simulink model "BuckyWagon_01"  (Simulink 7.5)
settings: Solver=FixedStepDiscrete  StartTime=0.0  StopTime=10.0  RelTol=1e-3
PreLoadFcn:
  | try, eval([bdroot '_setup']); catch, eval('model_setup', ''); end
InitFcn:
  | try, eval([bdroot '_setup']); catch, eval('model_setup', ''); end
undefined symbols (not defined in the file): ECU565, High, Low, miniviewSetup, motohawk_build_version, motohawk_get_faults, motohawk_setup_toolchains, motohawk_trunc_name, motohawk_vardec_config_group, motohawk_vardec_path, tc, True
libraries: MotoHawk_lib x381, simulink x26, miniview_lib x10, motohawk_control_primitives_lib x8, motohawk_engine_lib x6, motohawk_annotations_lib x2
(part 6 of 6)

== system BuckyWagon_01/Strategy/MiniViewDisplay/Send String_efficient/Subsystem ==
  string # : Inport  OutDataType=sfix(16)  OutScaling=2^0
  string : Inport  Port=2  OutDataType=sfix(16)  OutScaling=2^0
  Trigger : TriggerPort  TriggerType=function-call
  Demux3 : Demux  Outputs=[7 7 3 1]
  Function-Call Generator : simulink/Ports & Subsystems/Function-Call Generator  sample_time=-1  numberOfIterations=1
  Function-Call Subsystem : Subsystem  TreatAsAtomicUnit=on
  Function-Call Subsystem1 : Subsystem  TreatAsAtomicUnit=on
  Send Substring (page 0) : miniview_lib/Send Substring (page 0)  SystemSampleTime=-1  miniview_CAN_channel=miniview_CAN_channel
  Send Substring (page 1) : miniview_lib/Send Substring (page 1)  SystemSampleTime=-1  miniview_CAN_channel=miniview_CAN_channel
  Send Substring (page 2) : miniview_lib/Send Substring (page 2)  SystemSampleTime=-1  miniview_CAN_channel=miniview_CAN_channel
  Terminator : Terminator
  Terminator1 : Terminator
  wires:
  Demux3/3 -> Send Substring (page 2)/2
  Demux3/2 -> Send Substring (page 1)/2, Function-Call Subsystem1/1(In1)
  Demux3/1 -> Send Substring (page 0)/2, Function-Call Subsystem/1(In1)
  string/1 -> Demux3/1  "string"
  string #/1 -> Send Substring (page 1)/1, Send Substring (page 2)/1, Send Substring (page 0)/1  "string #"
  Function-Call Generator/1 -> Send Substring (page 0)/Trigger
  Send Substring (page 0)/1 -> Function-Call Subsystem/Trigger
  Function-Call Subsystem/1(Out) -> Send Substring (page 1)/Trigger
  Send Substring (page 1)/1 -> Function-Call Subsystem1/Trigger
  Function-Call Subsystem1/1(Out) -> Send Substring (page 2)/Trigger
  Demux3/4 -> Terminator/1
  Send Substring (page 2)/1 -> Terminator1/1

== system BuckyWagon_01/Strategy/MiniViewDisplay/Up Button/Subsystem ==
  Trigger : TriggerPort  TriggerType=function-call
  Read CAN Message : MotoHawk_lib/CAN Blocks/Read CAN Message  nam=['CAN_' num2str(miniview_CAN_channel)]  bus=-2  msg=miniview_button_up  queue=1  slot='miniview_button_up'  valid=off  stale=off  labelwires=on
  Signal Specification : SignalSpecification  DataType=boolean  OutDataType=sfix(16)  OutScaling=2^0  OutDataTypeStr=boolean
  Signal Specification1 : SignalSpecification  DataType=uint8  OutDataType=sfix(16)  OutScaling=2^0  OutDataTypeStr=uint8
  Up Asserted : Outport  OutDataType=sfix(16)  OutScaling=2^0
  Up Count : Outport  Port=2  OutDataType=sfix(16)  OutScaling=2^0
  wires:
  Signal Specification1/1 -> Up Count/1  "up count"
  Signal Specification/1 -> Up Asserted/1  "up asserted"
  Read CAN Message/2 -> Signal Specification1/1  "up count"
  Read CAN Message/1 -> Signal Specification/1  "up asserted"

== system BuckyWagon_01/Strategy/Sensors/Brusa Charger/PluggedInDetect ==
  MainsVolt : Inport  OutDataType=sfix(16)  OutScaling=2^0
  Thres : Inport  Port=2  OutDataType=sfix(16)  OutScaling=2^0
  Time : Inport  Port=3  OutDataType=sfix(16)  OutScaling=2^0
  Chart : Stateflow chart  TreatAsAtomicUnit=on
  Relational Operator : RelationalOperator  Operator=>  LogicOutDataTypeMode=boolean  OutDataTypeStr=boolean
  pluggedIn : Outport  OutDataType=sfix(16)  OutScaling=2^0
  wires:
  MainsVolt/1 -> Relational Operator/1
  Thres/1 -> Relational Operator/2
  Chart/1(pluggedIn) -> pluggedIn/1
  Relational Operator/1 -> Chart/2(mainsOn)
  Time/1 -> Chart/1(histTime)

== system BuckyWagon_01/Strategy/Sensors/Linear Sensor Characterization/If Action Subsystem ==
  In : Inport  OutDataType=sfix(16)  OutScaling=2^0
  Action Port : ActionPort  ActionType=then
  Out : Outport  OutDataType=sfix(16)  OutScaling=2^0
  wires:
  In/1 -> Out/1

== system BuckyWagon_01/Strategy/Sensors/Linear Sensor Characterization/If Action Subsystem1 ==
  In : Inport  OutDataType=sfix(16)  OutScaling=2^0
  Action Port : ActionPort  ActionType=elseif
  Out : Outport  OutDataType=sfix(16)  OutScaling=2^0
  wires:
  In/1 -> Out/1

== system BuckyWagon_01/Strategy/Sensors/Linear Sensor Characterization/If Action Subsystem2 ==
  In : Inport  OutDataType=sfix(16)  OutScaling=2^0
  Action Port : ActionPort  ActionType=else
  Out : Outport  OutDataType=sfix(16)  OutScaling=2^0
  wires:
  In/1 -> Out/1

== system BuckyWagon_01/Strategy/Control Strategy/Assist/StallTorqueFault/Hysterisis ==
  HiThresh : Inport  OutDataType=sfix(16)  OutScaling=2^0
  LowThresh : Inport  Port=2  OutDataType=sfix(16)  OutScaling=2^0
  Signal : Inport  Port=3  OutDataType=sfix(16)  OutScaling=2^0
  Hysteresis : Subsystem
  LT : RelationalOperator  ZeroCross=off  InputSameDT=on
  LT1 : RelationalOperator  Operator=<=  ZeroCross=off  InputSameDT=on
  Threshold : Outport  OutDataType=sfix(16)  OutScaling=2^0
  wires:
  LT/1 -> Hysteresis/1(Hi)  "AboveHiTarget"
  LT1/1 -> Hysteresis/2(Lo)  "BelowLoTarget"
  Hysteresis/1("Out (Lo=0, Hi=1)") -> Threshold/1
  HiThresh/1 -> LT/2
  LowThresh/1 -> LT1/2
  Signal/1 -> LT/1, LT1/1

== system BuckyWagon_01/Strategy/Control Strategy/HV Controller/Contacter Controller/Delay ==
  note: Delay the rising and falling of a boolean signal
  In : Inport  OutDataType=sfix(16)  OutScaling=2^0
  Constant1 : Constant  Value=0  OutDataType=sfix(16)  OutScaling=2^0  OutDataTypeStr=Inherit: Inherit via back propagation
  Constant3 : Constant  Value=0  OutDataType=sfix(16)  OutScaling=2^0  OutDataTypeStr=Inherit: Inherit via back propagation
  Data Type Conversion : DataTypeConversion  OutDataType=sfix(16)  OutScaling=2^0  RndMeth=Zero
  Data Type Conversion1 : DataTypeConversion  OutDataType=sfix(16)  OutScaling=2^0  RndMeth=Zero
  Logical Operator : Logic  Operator=NOT  OutDataTypeMode=boolean  OutDataTypeStr=boolean
  Logical Operator1 : Logic  OutDataTypeMode=boolean  OutDataTypeStr=boolean
  Logical Operator2 : Logic  OutDataTypeMode=boolean  OutDataTypeStr=boolean
  MotoHawk S-R Flip-Flop : Subsystem  mask(MotoHawk S-R Flip-Flop){ic_bool=false}
      mask prompts: ic_bool "Initial condition Q (boolean)"
      mask help:
      | When input S (set) is TRUE, output Q is TRUE (and latched until reset).
      | When input R (reset) is TRUE, output Q is FALSE (and latched until set).
      | If both inputs S and R are TRUE, output Q is FALSE (reset wins).
      mask Display:
      | patch([0 0 1 1], [0 0.075 0.075 0], [230/255 0/255 0/255])
      | patch([0 0 1 1], [0.025 0.05 0.05 0.025], [150/255 0/255 0/255])
      | patch([0 0 1 1], [0 0.025 0.025 0], [0/255 0/255 0/255])
  Relational Operator1 : RelationalOperator  LogicOutDataTypeMode=boolean  OutDataTypeStr=boolean  ZeroCross=off  InputSameDT=on
  Relational Operator2 : RelationalOperator  LogicOutDataTypeMode=boolean  OutDataTypeStr=boolean  ZeroCross=off  InputSameDT=on
  Sum : Sum  Inputs=++|  OutDataType=sfix(16)  OutScaling=2^0  RndMeth=Zero  SaturateOnIntegerOverflow=on  InputSameDT=on
  Sum1 : Sum  Inputs=++|  OutDataType=sfix(16)  OutScaling=2^0  RndMeth=Zero  SaturateOnIntegerOverflow=on  InputSameDT=on
  Switch : Switch  Criteria=u2 ~= 0  Threshold=1  RndMeth=Zero  ZeroCross=off  InputSameDT=on
  Switch1 : Switch  Criteria=u2 ~= 0  Threshold=1  RndMeth=Zero  ZeroCross=off  InputSameDT=on
  Terminator : Terminator
  Unit Delay : UnitDelay  SampleTime=-1
  Unit Delay1 : UnitDelay  SampleTime=-1
  off delay : Constant  Value=10  OutDataType=sfix(16)  OutScaling=2^0
  on delay : Constant  Value=0  OutDataType=sfix(16)  OutScaling=2^0
  Out : Outport  OutDataType=sfix(16)  OutScaling=2^0
  wires:
  Logical Operator1/1 -> MotoHawk S-R Flip-Flop/2(R)
  Logical Operator2/1 -> MotoHawk S-R Flip-Flop/1(S)
  Relational Operator1/1 -> Logical Operator2/2
  Relational Operator2/1 -> Logical Operator1/2
  MotoHawk S-R Flip-Flop/2(!Q) -> Terminator/1
  MotoHawk S-R Flip-Flop/1(Q) -> Out/1
  off delay/1 -> Relational Operator2/2
  Logical Operator/1 -> Logical Operator1/1, Switch1/2, Data Type Conversion1/1
  Data Type Conversion1/1 -> Sum1/2  "0 to 1"
  Sum1/1 -> Switch1/1  "0 to 65535 (saturate hi)"
  Constant3/1 -> Switch1/3
  Switch1/1 -> Relational Operator2/1, Unit Delay1/1  "0 to 65535"
  In/1 -> Logical Operator/1, Logical Operator2/1, Switch/2, Data Type Conversion/1
  Data Type Conversion/1 -> Sum/2  "0 to 1"
  Sum/1 -> Switch/1  "0 to 65535 (saturate hi)"
  Constant1/1 -> Switch/3
  Switch/1 -> Unit Delay/1, Relational Operator1/1  "0 to 65535"
  on delay/1 -> Relational Operator1/2
  Unit Delay1/1 -> Sum1/1  "0 to 65535"
  Unit Delay/1 -> Sum/1  "0 to 65535"

== system BuckyWagon_01/Strategy/MiniViewDisplay/Send String_efficient/Subsystem/Function-Call Subsystem ==
  In1 : Inport  OutDataType=sfix(16)  OutScaling=2^0
  function : TriggerPort  TriggerType=function-call
  Compare To Zero : simulink/Logic and Bit Operations/Compare To Zero  SystemSampleTime=-1  relop=~=  LogicOutDataTypeMode=uint8  ZeroCross=off
  Enabled Subsystem : Subsystem  TreatAsAtomicUnit=on
  Logical Operator : Logic  Inputs=1  AllPortsSameDT=off  OutDataTypeMode=boolean  OutDataTypeStr=boolean
  Out : Outport  OutDataType=sfix(16)  OutScaling=2^0
  wires:
  Compare To Zero/1 -> Logical Operator/1
  In1/1 -> Compare To Zero/1
  Logical Operator/1 -> Enabled Subsystem/Enable
  Enabled Subsystem/1(Out1) -> Out/1

== system BuckyWagon_01/Strategy/MiniViewDisplay/Send String_efficient/Subsystem/Function-Call Subsystem1 ==
  In1 : Inport  OutDataType=sfix(16)  OutScaling=2^0
  function : TriggerPort  TriggerType=function-call
  Compare To Zero : simulink/Logic and Bit Operations/Compare To Zero  SystemSampleTime=-1  relop=~=  LogicOutDataTypeMode=uint8  ZeroCross=off
  Enabled Subsystem : Subsystem  TreatAsAtomicUnit=on
  Logical Operator : Logic  Inputs=1  AllPortsSameDT=off  OutDataTypeMode=boolean  OutDataTypeStr=boolean
  Out : Outport  OutDataType=sfix(16)  OutScaling=2^0
  wires:
  Enabled Subsystem/1(Out1) -> Out/1
  Logical Operator/1 -> Enabled Subsystem/Enable
  In1/1 -> Compare To Zero/1
  Compare To Zero/1 -> Logical Operator/1

== system BuckyWagon_01/Strategy/Control Strategy/Assist/StallTorqueFault/Hysterisis/Hysteresis ==
  note: Hi & !Lo => Hi
      | Lo & !Hi => Lo
      | Otherwise, Hold
  Hi : Inport  OutDataType=sfix(16)  OutScaling=2^0
  Lo : Inport  Port=2  OutDataType=sfix(16)  OutScaling=2^0
  Combinatorial  Logic : CombinatorialLogic  TruthTable=[0 0;0 1;1 1;0 0]
  Demux : Demux  Outputs=2
  Mux : Mux  Inputs=2
  Switch1 : Switch  Threshold=0.5  SaturateOnIntegerOverflow=on  InputSameDT=on
  Unit Delay : UnitDelay  SampleTime=-1
  "Out (Lo=0, Hi=1)" : Outport  OutDataType=sfix(16)  OutScaling=2^0
  wires:
  Mux/1 -> Combinatorial  Logic/1
  Combinatorial  Logic/1 -> Demux/1
  Demux/1 -> Switch1/1
  Demux/2 -> Switch1/2
  Unit Delay/1 -> Switch1/3
  Switch1/1 -> Unit Delay/1, "Out (Lo=0, Hi=1)"/1
  Hi/1 -> Mux/1
  Lo/1 -> Mux/2

== system BuckyWagon_01/Strategy/Control Strategy/HV Controller/Contacter Controller/Delay/MotoHawk S-R Flip-Flop ==
  note: MotoHawk S-R Flip-Flop
  S : Inport  OutDataType=sfix(16)  OutScaling=2^0
  R : Inport  Port=2  OutDataType=sfix(16)  OutScaling=2^0
  Logical Operator : Logic  Operator=OR  OutDataTypeMode=boolean  OutDataTypeStr=boolean
  Logical Operator1 : Logic  Operator=NOT  OutDataTypeMode=boolean  OutDataTypeStr=boolean
  Logical Operator2 : Logic  OutDataTypeMode=boolean  OutDataTypeStr=boolean
  Logical Operator3 : Logic  Operator=NOT  OutDataTypeMode=boolean  OutDataTypeStr=boolean
  Signal Specification : SignalSpecification  DataType=boolean  OutDataType=sfix(16)  OutScaling=2^0  OutDataTypeStr=boolean
  Signal Specification1 : SignalSpecification  DataType=boolean  OutDataType=sfix(16)  OutScaling=2^0  OutDataTypeStr=boolean
  Unit Delay : UnitDelay  X0=ic_bool  SampleTime=-1
  Q : Outport  OutDataType=sfix(16)  OutScaling=2^0
  !Q : Outport  Port=2  OutDataType=sfix(16)  OutScaling=2^0
  wires:
  Logical Operator3/1 -> !Q/1
  R/1 -> Signal Specification/1
  S/1 -> Signal Specification1/1
  Signal Specification1/1 -> Logical Operator/2
  Signal Specification/1 -> Logical Operator1/1
  Logical Operator2/1 -> Q/1, Unit Delay/1, Logical Operator3/1
  Unit Delay/1 -> Logical Operator/1
  Logical Operator/1 -> Logical Operator2/1
  Logical Operator1/1 -> Logical Operator2/2

== system BuckyWagon_01/Strategy/MiniViewDisplay/Send String_efficient/Subsystem/Function-Call Subsystem/Enabled Subsystem ==
  Enable : EnablePort
  Function-Call Generator : simulink/Ports & Subsystems/Function-Call Generator  sample_time=-1  numberOfIterations=1
  Out1 : Outport  OutDataType=sfix(16)  OutScaling=2^0
  wires:
  Function-Call Generator/1 -> Out1/1

== system BuckyWagon_01/Strategy/MiniViewDisplay/Send String_efficient/Subsystem/Function-Call Subsystem1/Enabled Subsystem ==
  Enable : EnablePort
  Function-Call Generator : simulink/Ports & Subsystems/Function-Call Generator  sample_time=-1  numberOfIterations=1
  Out1 : Outport  OutDataType=sfix(16)  OutScaling=2^0
  wires:
  Function-Call Generator/1 -> Out1/1

== stateflow chart Strategy/Control Strategy/Reverse/Chart ==
  state Main
    state ButtonDebounce [parallel]
      settings: executionOrder=1
      state waitRelease
        entry:buttonPress;
      state TransistionOn
        during:timer++;
      state TransistionOff
        during:timer++;
      TransistionOff -> TransistionOff [order 2] : [revButton]
          | {timer = 0;}
      TransistionOff -> TransistionOn [order 1] : [timer >= offTime]
      TransistionOn -> waitRelease [order 2] : [timer >= onTime]
      waitRelease -> TransistionOff : [~revButton]
      TransistionOn -> TransistionOn [order 1] : [~revButton]
          | {timer = 0;}
      (default) -> TransistionOn
    state ReverseLogic [parallel]
      settings: executionOrder=2
      state Forward
        entry:inReverse = 0;
      state Reverse
        entry:inReverse = 1;
      Reverse -> Forward : buttonPress...
          | [(speed < fwdSpdThres)&&...
          | (accel < fwdAccThres)]
      Forward -> Reverse : buttonPress...
          | [(speed < revSpdThres)&&...
          | (accel < revAccThres)]
      (default) -> Forward
  data: accel input double; speed input double; revButton input double; fwdAccThres input double; fwdSpdThres input double; inReverse output double; offTime input double; revAccThres input double; revSpdThres input double; timer local double; onTime input double
  events: buttonPress local EITHER_EDGE_EVENT

== stateflow chart Strategy/MiniViewDisplay/Chart ==
  state List
    state List_Wait
    state List_Wait2
    state List_Idle
      entry:
      stringNum = 0;
    state List_Init
      entry:
      clearScreen;
      //draw lines and name
      stringNum = 15;
      sprintf(charPtr(&string[0]), "UWMAD");
      string[5] = 0;
      sendString;
      y0 = 8;
      x0 = 0;
      x1 = 63;
      lineColor = BLACK;
      fillColor = WHITE;
      drawHLine;
      y0 = 54;
      drawHLine;
      hCenter = 1;
      vCenter = 0;
      font = FONT4x6;
      x0 = 32;
      y0 = 2;
      drawString;
      listIndexO = listIndex;
    (junction 83) -> (junction 93) [order 1] : [statusTxtMode == 1]...
        | {fillColor = BLACK; lineColor = BLACK;...
        | drawRect; lineColor = WHITE;}
    (junction 90) -> (junction 83) [order 2] : {y0 = 55; y1 = 63; x0 = 0; x1 = 63;...
        | memcpy(&string[0], &statusTxt[0], 9);...
        | string[9] = 0; sendString;}
    (junction 83) -> (junction 93) [order 2] : {lineColor = WHITE;...
        | drawRect;...
        | lineColor = BLACK;}
    List.List_Idle -> List.List_Idle [order 2] : tick /timer++;
    (junction 85) -> List.List_Idle : {timer = 0;}
    (junction 86) -> List.List_Idle [order 1] : [listIndex == 0]
    List.List_Idle -> (junction 86) [order 3] : upPressed
    (junction 86) -> (junction 87) [order 2] : {listIndexO = listIndex-1;...
        | writeListIndex;}
    List_Init -> (junction 87)
    List.List_Idle -> (junction 88) [order 4] : downPressed
    (junction 88) -> (junction 87) [order 2] : {listIndexO = listIndex+1;...
        | writeListIndex;;}
    (junction 88) -> List.List_Idle [order 1] : [listIndex == numFields-6]
    (junction 93) -> (junction 85) : {y0 = 56; font = FONT4x6; x0 = 17;...
        | drawString;}
    (junction 89) -> (junction 90) [order 2] : {sprintf(charPtr(&string[0]), "%-4d", data[stringNum+listIndex]);...
        | string[4] = 0; sendString;...
        | x0 = 42; x1 = 57; y0 = 12+stringNum*7; y1 = y0+6;...
        | lineColor = 0; drawRect; lineColor = 1
        | drawString;...
        |  oldData[stringNum] = data[stringNum+listIndex];...
        | stringNum++;}
    List.List_Idle -> (junction 90) [order 1] : tick [timer >= UPDATE_TIME]...
        | {stringNum = 0;...
        | fillColor = WHITE; hCenter = 0;}
    (junction 90) -> (junction 89) [order 1] : [stringNum < 6]
    (junction 87) -> (junction 91) : {stringNum = 0;}
    (junction 89) -> (junction 90) [order 1] : [oldData[stringNum] == data[stringNum+listIndex]]...
        | {stringNum++;}
    (junction 91) -> (junction 91) [order 1] : [stringNum < 6]...
        | {memcpy(&string[0], &names[10*(listIndexO+stringNum)], 10);...
        | sendString; stringNum++;}
    List_Wait2 -> (junction 90) : {stringNum = 0;}
    (junction 91) -> List_Wait [order 2]
    (junction 121) -> List_Init [order 2]
    (junction 92) -> List_Wait2 [order 2]
    List_Wait -> (junction 92) : {x0 = 9; y0 = 12; x1 = 41; y1 = 53;
        | lineColor = 0; fillColor = 0;
        | drawRect; lineColor = 1;
        | hCenter = 0; stringNum = 0;}
    (junction 121) -> (junction 121) [order 1] : [stringNum < 6]...
        | {oldData[stringNum] = ...
        | data[stringNum+listIndex]+1;...
        | stringNum++;}
    (junction 92) -> (junction 92) [order 1] : [stringNum < 6]...
        | {y0 = 12 + stringNum*7;...
        | drawString;stringNum++;}
    (default) -> (junction 121) : {stringNum = 0}
  state PowerupDelay
    entry:timer = 0;
    during:timer++;
  state Single
    state singleNames
      entry:
      hCenter = 1;
      font = FONT6x8;
      x0 = 30;
      stringNum = 0;
      memcpy(&string[0], &names[10*singleIndex], 10);
      sendString;
      y0 = 14;
      drawString;
    state Single_Init
      entry:
      clearScreen;
      //draw string
      stringNum = 15;
      sprintf(charPtr(&string[0]), "UWMAD");
      string[5] = 0;
      sendString;
      hCenter = 1;
      vCenter = 0;
      font = FONT4x6;
      x0 = 32; y0 = 2;
      lineColor = BLACK;
      fillColor = WHITE;
      drawString;
      //draw lines
      y0 = 8; x0 = 0; x1 = 64;
      drawHLine;
      y0 = 54;
      drawHLine;
      oldData[0] = data[singleIndex]+1
    state List_Idle
    (junction 76) -> (junction 74) : {y0 = 56; font = FONT4x6; x0 = 17;...
        | drawString;}
    (junction 117) -> (junction 118) [order 4] : [barGraphMode[singleIndex] == 3]...
        | {x0 = temp;...
        | drawVLine;}
    Single_Init -> singleNames
    (default) -> Single_Init
    (junction 75) -> (junction 76) [order 1] : [statusTxtMode == 1]...
        | {fillColor = BLACK; lineColor = BLACK;...
        | drawRect; lineColor = WHITE;}
    (junction 119) -> (junction 75) : {y0 = 55; y1 = 63; x0 = 0; x1 = 63;...
        | memcpy(&string[0], &statusTxt[0], 9);...
        | string[9] = 0; sendString;}
    (junction 120) -> (junction 119)
    (junction 74) -> Single.List_Idle : {timer = 0;}
    Single.List_Idle -> Single.List_Idle [order 2] : tick /timer++;
    (junction 115) -> (junction 119) [order 1] : [oldData[0] ==...
        |  data[singleIndex] ]
    (junction 118) -> (junction 120)
    (junction 117) -> (junction 118) [order 3] : [barGraphMode[singleIndex] == 1]...
        | {x0 = temp; fillColor = BLACK; drawRect;}
    (junction 116) -> (junction 117) [order 3] : {temp = (int32(data[singleIndex]) - barMin[singleIndex] )*52 /...
        |  (barMax[singleIndex]-barMin[singleIndex]) + 6;}
    (junction 117) -> (junction 118) [order 2] : [(barGraphMode[singleIndex] == 2) && (temp < 32)]...
        | {x0 = temp; x1 = 32; fillColor = BLACK; drawRect;}
    Single.List_Idle -> (junction 115) [order 1] : tick [timer >= UPDATE_TIME]...
        | {stringNum = 0;font = FONT8x15;...
        | fillColor = WHITE; hCenter = 0;}
    (junction 117) -> (junction 118) [order 5] : {x1 = temp; fillColor = BLACK; drawRect;}
    (junction 116) -> (junction 117) [order 2] : [data[singleIndex] <min(barMin[singleIndex], barMax[singleIndex])]...
        | {temp = ((min(barMin[singleIndex], barMax[singleIndex]) -...
        | barMin[singleIndex] )*52 / (barMax[singleIndex]-barMin[singleIndex])) + 6;}
    (junction 115) -> (junction 116) [order 2] : {sprintf(charPtr(&string[0]), "%4d", data[singleIndex]);...
        | sendString;...
        | x0 = 0; x1 = 64; y0 = 25; y1 = 39;fillColor = WHITE;...
        | lineColor = 0; drawRect; lineColor = BLACK; x0 = 15;...
        | drawString; oldData[0] = data[singleIndex];
        | x0 = 6; x1 = 58; y0 = 41; y1 = 48;
        | lineColor = BLACK; drawRect;}
    (junction 116) -> (junction 117) [order 1] : [data[singleIndex] > max(barMin[singleIndex], barMax[singleIndex])]...
        | {temp = ((max(barMin[singleIndex], barMax[singleIndex]) - ...
        | barMin[singleIndex] )*52 / (barMax[singleIndex]-barMin[singleIndex])) + 6;}
    (junction 117) -> (junction 118) [order 1] : [(barGraphMode[singleIndex] == 2) && (temp >= 32)]...
        | {x1 = temp; fillColor = BLACK; x0 = 32; drawRect;}
    singleNames -> Single.List_Idle : {timer = UPDATE_TIME;}
    (junction 75) -> (junction 76) [order 2] : {lineColor = WHITE;...
        | fillColor = WHITE;...
        | drawRect;...
        | lineColor = BLACK;}
  state Setup
    state wait
      entry:
      clearScreen;
      setupIndex = 0;
    state setup_Wait
    state setup_Idle
      entry:
      stringNum = 0;
    state Setup_Init
      entry:
      clearScreen;
      //draw lines and name
      stringNum = 15;
      sprintf(charPtr(&string[0]), "UWMAD");
      string[5] = 0;
      sendString;
      y0 = 8;
      x0 = 0;
      x1 = 63;
      lineColor = BLACK;
      fillColor = WHITE;
      drawHLine;
      y0 = 54;
      drawHLine;
      hCenter = 1;
      vCenter = 0;
      font = FONT4x6;
      x0 = 32;
      y0 = 2;
      drawString;
      setupVIndex = 0;
    state storeSelect [function]
      (junction 102) -> (junction 103) [order 1] : [setupIndex == 1]...
          | {singleIndexO = selectIndex; writeSingleIndex;}
      (default) -> (junction 102)
      (junction 102) -> (junction 103) [order 2] : [(setupIndex == 2) || (setupIndex == 3)]...
          | {dualIndexO = dualIndex;...
          | dualIndexO[setupIndex-2] = selectIndex;...
          | writeDualIndex;}
      (junction 102) -> (junction 103) [order 3] : [setupIndex >= 4]...
          | {quadIndexO = quadIndex;...
          | quadIndexO[setupIndex-4] = selectIndex;...
          |  writeQuadIndex;}
    state loadSelect [function]
      (junction 100) -> (junction 101) [order 1] : [setupIndex == 1]...
          | {selectIndex = singleIndex;}
      (default) -> (junction 100)
      (junction 100) -> (junction 101) [order 2] : [(setupIndex == 2) || (setupIndex == 3)]...
          | {selectIndex = dualIndex[setupIndex-2];}
      (junction 100) -> (junction 101) [order 3] : [setupIndex >= 4]...
          | {selectIndex = quadIndex[setupIndex-4];}
    state select_var
      state select_Wait
      state select_Idle
        entry:
      state Select_Init
        entry:
        clearScreen;
        //draw lines and name
        stringNum = 15;
        sprintf(charPtr(&string[0]), "UWMAD");
        string[5] = 0;
        sendString;
        y0 = 8;
        x0 = 0;
        x1 = 63;
        lineColor = BLACK;
        fillColor = WHITE;
        drawHLine;
        y0 = 54;
        drawHLine;
        hCenter = 1;
        vCenter = 0;
        font = FONT4x6;
        x0 = 32;
        y0 = 2;
        drawString;
        selectIndex = 0;
        selectVIndex = 0;
      (junction 94) -> (junction 95) [order 1] : [stringNum < 6]...
          | {y0 = 12 + stringNum*7;}
      (junction 96) -> (junction 96) [order 1] : [stringNum < 6]...
          | {memcpy(&string[0], &names[10*(selectVIndex+stringNum)], 10);...
          | sendString; stringNum++;}
      (junction 95) -> (junction 94) [order 1] : [(selectVIndex+stringNum) == selectIndex]...
          | {fillColor = BLACK; lineColor = WHITE;...
          | drawString;stringNum++;}
      select_Wait -> (junction 94) : {x0 = 0; y0 = 12; x1 = 64; y1 = 53;
          | lineColor = 0; fillColor = 0;
          | drawRect; lineColor = 1;
          | hCenter = 1; stringNum = 0;}
      (junction 95) -> (junction 94) [order 2] : {fillColor = WHITE; lineColor = BLACK;...
          | drawString;stringNum++;}
      (junction 96) -> select_Wait [order 2]
      (junction 94) -> select_Idle [order 2]
      (junction 98) -> (junction 96) [order 2] : [selectIndex < selectVIndex]...
          | {selectVIndex = selectIndex;...
          | stringNum = 0;}
      (junction 98) -> (junction 96) [order 1] : [selectIndex >= (selectVIndex +6)]...
          | {selectVIndex = selectIndex -5;
          | stringNum = 0;}
      (junction 98) -> (junction 96) [order 3] : {stringNum = 0;}
      (default) -> Select_Init
      (junction 97) -> select_Idle [order 1] : [selectIndex ==...
          |  (numFields-1)]
      (junction 97) -> (junction 98) [order 2] : {selectIndex++;}
      select_Idle -> (junction 97) [order 3] : downPressed
      Select_Init -> (junction 98)
      (junction 99) -> (junction 98) [order 2] : {selectIndex--;}
      select_Idle -> (junction 99) [order 2] : upPressed
      (junction 99) -> select_Idle [order 1] : [selectIndex == 0]
    (junction 67) -> (junction 68) [order 1] : [stringNum < 6]...
        | {y0 = 12 + stringNum*7;}
    (junction 69) -> (junction 69) [order 1] : [stringNum < 6]...
        | {memcpy(&string[0], &setupNames[13*(setupVIndex+stringNum)], 13);...
        | sendString; stringNum++;}
    (junction 68) -> (junction 67) [order 1] : [(setupVIndex+stringNum) == setupIndex]...
        | {fillColor = BLACK; lineColor = WHITE;...
        | drawString;stringNum++;}
    setup_Wait -> (junction 67) : {x0 = 0; y0 = 12; x1 = 64; y1 = 53;
        | lineColor = 0; fillColor = 0;
        | drawRect; lineColor = 1;
        | hCenter = 1; stringNum = 0;}
    (junction 68) -> (junction 67) [order 2] : {fillColor = WHITE; lineColor = BLACK;...
        | drawString;stringNum++;}
    (junction 69) -> setup_Wait [order 2]
    (junction 67) -> setup_Idle [order 2]
    (junction 71) -> (junction 69) [order 2] : [setupIndex < setupVIndex]...
        | {setupVIndex = setupIndex;...
        | stringNum = 0;}
    (junction 71) -> (junction 69) [order 1] : [setupIndex >= (setupVIndex +6)]...
        | {setupVIndex = setupIndex -5;
        | stringNum = 0;}
    (junction 71) -> (junction 69) [order 3] : {stringNum = 0;}
    (junction 70) -> setup_Idle [order 1] : [setupIndex == 7]
    (junction 70) -> (junction 71) [order 2] : {setupIndex++;}
    setup_Idle -> (junction 70) [order 3] : downPressed
    Setup_Init -> (junction 71)
    (junction 72) -> (junction 71) [order 2] : {setupIndex--;}
    setup_Idle -> (junction 72) [order 2] : upPressed
    (junction 72) -> setup_Idle [order 1] : [setupIndex == 0]
    select_Idle -> Setup_Init [order 1] : menuReleased...
        | {storeSelect();}
    setup_Idle -> (junction 73) [order 1] : menuReleased
    (junction 73) -> select_var [order 2] : {loadSelect();}
    wait -> Setup_Init : menuReleased
    (default) -> wait
  state wait1
  state Dual
    state List_Idle
    state dualNames
      entry:
      hCenter = 1;
      font = FONT6x8; x0 = 30;
      stringNum = 0;
      memcpy(&string[0], &names[10*dualIndex[0]], 10);
      sendString;
      y0 = 20;drawString;
      memcpy(&string[0], &names[10*dualIndex[1]], 10);
      sendString;
      y0 = 34;drawString;
    state Dual_Init
      entry:
      clearScreen;
      //draw string
      stringNum = 15;
      sprintf(charPtr(&string[0]), "UWMAD");
      string[5] = 0;
      sendString;
      hCenter = 1;
      vCenter = 0;
      font = FONT4x6;
      x0 = 32; y0 = 2;
      lineColor = BLACK;
      fillColor = WHITE;
      drawString;
      //draw lines
      y0 = 8; x0 = 0; x1 = 64;
      drawHLine;
      y0 = 54;
      drawHLine;
      y0 = 31;
      drawHLine;
    (junction 114) -> (junction 78) : {y0 = 55; y1 = 63; x0 = 0; x1 = 63;...
        | memcpy(&string[0], &statusTxt[0], 9);...
        | string[9] = 0; sendString;}
    (junction 77) -> Dual.List_Idle : {timer = 0;}
    (junction 113) -> (junction 114) [order 1] : [oldData[1] ==...
        |  data[dualIndex[1]] ]
    (junction 78) -> (junction 79) [order 2] : {lineColor = WHITE;...
        | drawRect;...
        | lineColor = BLACK;}
    (junction 79) -> (junction 77) : {y0 = 56; font = FONT4x6; x0 = 17;...
        | drawString;}
    (junction 78) -> (junction 79) [order 1] : [statusTxtMode == 1]...
        | {fillColor = BLACK; lineColor = BLACK;...
        | drawRect; lineColor = WHITE;}
    (default) -> (junction 111) : {stringNum = 0}
    (junction 111) -> (junction 111) [order 1] : [stringNum < 2]...
        | {oldData[stringNum] = ...
        | data[dualIndex[stringNum]]+1;...
        | stringNum++;}
    (junction 111) -> Dual_Init [order 2]
    Dual_Init -> dualNames
    dualNames -> Dual.List_Idle : {timer = UPDATE_TIME;}
    Dual.List_Idle -> (junction 112) [order 1] : tick [timer >= UPDATE_TIME]...
        | {stringNum = 0; font = FONT6x8;...
        | fillColor = WHITE; hCenter = 0;}
    (junction 112) -> (junction 113) [order 2] : {sprintf(charPtr(&string[0]), "%d", data[dualIndex[0]]);...
        | sendString;...
        | x0 = 0; x1 = 60; y0 = 10; y1 = 18;...
        | lineColor = 0; drawRect; lineColor = 1; x0 = 30;...
        | drawString; oldData[0] = data[dualIndex[0]];}
    (junction 112) -> (junction 113) [order 1] : [oldData[0] ==...
        |  data[dualIndex[0]] ]
    Dual.List_Idle -> Dual.List_Idle [order 2] : tick /timer++;
    (junction 113) -> (junction 114) [order 2] : {sprintf(charPtr(&string[0]), "%d", data[dualIndex[1]]);...
        | sendString;...
        | x0 = 0; x1 = 60; y0 = 44; y1 = 53;...
        | lineColor = 0; drawRect; lineColor = 1; x0 = 30;...
        | drawString; oldData[1] = data[dualIndex[1]];}
  state Quad
    state Quad_Idle
    state Quad_Init
      entry:
      clearScreen;
      //draw string
      stringNum = 15;
      sprintf(charPtr(&string[0]), "UWMAD");
      string[5] = 0;
      sendString;
      hCenter = 1;
      vCenter = 0;
      font = FONT4x6;
      x0 = 32; y0 = 2;
      lineColor = BLACK;
      fillColor = WHITE;
      drawString;
      //draw lines
      y0 = 8; x0 = 0; x1 = 64;
      drawHLine;
      y0 = 54;
      drawHLine;
      y0 = 31;
      drawHLine;
      y0 = 8; y1 = 54; x0 = 30;;
      drawVLine;
    state Quad_Names
      entry:
      hCenter = 0;
      x0 = 10; y0 = 10; stringNum = 0; drawString;
      x0 = 5; y0 = 16; stringNum = 4; drawString;
      y0 = 41; stringNum = 2; drawString;
      x0 = 10; y0 = 47; stringNum = 6; drawString;
      x0 = 32; y0 = 10; stringNum = 1; drawString;
      y0 = 16; stringNum = 5; drawString;
      y0 = 41; stringNum = 3; drawString;
      y0 = 47; stringNum = 7; drawString;
    (junction 82) -> (junction 80) : {y0 = 56; font = FONT4x6; x0 = 17;...
        | drawString;}
    (junction 81) -> (junction 82) [order 2] : {lineColor = WHITE;...
        | drawRect;...
        | lineColor = BLACK;}
    (junction 110) -> (junction 81) : {y0 = 55; y1 = 63; x0 = 0; x1 = 63;...
        | memcpy(&string[0], &statusTxt[0], 9);...
        | string[9] = 0; sendString;}
    (junction 81) -> (junction 82) [order 1] : [statusTxtMode == 1]...
        | {fillColor = BLACK; lineColor = BLACK;...
        | drawRect; lineColor = WHITE;}
    (junction 104) -> (junction 104) [order 1] : [stringNum < 4]...
        | {memcpy(&string[0], &namesline1[7*quadIndex[stringNum]], 7);...
        | sendString;...
        | memcpy(&string[0], &namesline2[7*quadIndex[stringNum]], 7);...
        | stringNum = stringNum+4; sendString; stringNum = stringNum-3;...
        | }
    (junction 104) -> Quad_Names [order 2]
    Quad_Init -> (junction 104) : {stringNum = 0;}
    (default) -> (junction 105) : {stringNum = 0}
    Quad_Names -> Quad_Idle : {timer = UPDATE_TIME;...
        | font = FONT6x8;}
    (junction 105) -> (junction 105) [order 1] : [stringNum < 4]...
        | {oldData[stringNum] = ...
        | data[quadIndex[stringNum]]+1;...
        | stringNum++;}
    (junction 105) -> Quad_Init [order 2]
    Quad_Idle -> (junction 106) [order 1] : tick [timer >= UPDATE_TIME]...
        | {stringNum = 0; font = FONT6x8;...
        |  fillColor = WHITE; hCenter = 0;}
    (junction 106) -> (junction 107) [order 2] : {sprintf(charPtr(&string[0]),"%4d", data[quadIndex[0]]);...
        | sendString;...
        | x0 = 5; x1 = 29; y0 = 23; y1 = 30;...
        | lineColor = 0; drawRect; lineColor = 1;...
        | drawString; oldData[0] = data[quadIndex[0]];}
    (junction 106) -> (junction 107) [order 1] : [oldData[0] ==...
        |  data[quadIndex[0]] ]
    Quad_Idle -> Quad_Idle [order 2] : tick /timer++;
    (junction 107) -> (junction 108) [order 2] : {sprintf(charPtr(&string[0]), "%-4d", data[quadIndex[1]]);...
        | sendString;...
        | x0 = 32; x1 = 55; y0 = 23; y1 = 30;...
        | lineColor = 0; drawRect; lineColor = 1;...
        | drawString; oldData[1] = data[quadIndex[1]];}
    (junction 107) -> (junction 108) [order 1] : [oldData[1] ==...
        |  data[quadIndex[1]] ]
    (junction 108) -> (junction 109) [order 2] : {sprintf(charPtr(&string[0]), "%4d", data[quadIndex[2]]);...
        | sendString;...
        | x0 = 5; x1 = 29; y0 = 33; y1 = 40;...
        | lineColor = 0; drawRect; lineColor = 1;...
        | drawString; oldData[2] = data[quadIndex[2]];}
    (junction 108) -> (junction 109) [order 1] : [oldData[2] ==...
        |  data[quadIndex[2]] ]
    (junction 80) -> Quad_Idle : {timer = 0;}
    (junction 109) -> (junction 110) [order 2] : {sprintf(charPtr(&string[0]), "%-4d", data[quadIndex[3]]);...
        | sendString;...
        | x0 = 32; x1 = 55; y0 = 33; y1 = 40;...
        | lineColor = 0; drawRect; lineColor = 1;...
        | drawString; oldData[3] = data[quadIndex[3]];}
    (junction 109) -> (junction 110) [order 1] : [oldData[3] ==...
        |  data[quadIndex[3]] ]
  state wait4
  state wait3
  state wait2
  wait3 -> Setup [order 2] : [menuTime >= SETUP_TIME]
  (junction 84) -> Single [order 1] : [screen == 1]
  wait2 -> Setup [order 2] : [menuTime >= SETUP_TIME]
  (junction 84) -> Quad [order 3] : [screen == 3]
  wait4 -> Setup [order 2] : [menuTime >= SETUP_TIME]
  PowerupDelay -> (junction 84) : [timer >= startupDelay]
  (junction 84) -> List [order 4]
  (junction 84) -> Dual [order 2] : [screen == 2]
  (default) -> PowerupDelay
  List -> wait4 : menuPressed
  (junction 73) -> (junction 84) [order 1] : [setupIndex == 0]
  Single -> wait3 : menuPressed
  Dual -> wait2 : menuPressed
  Quad -> wait1 : menuPressed
  wait1 -> Setup [order 2] : [menuTime >= SETUP_TIME]
  wait4 -> Quad [order 1] : menuReleased...
      | {screenO = 4; writeScreen;}
  wait3 -> List [order 1] : menuReleased...
      | {screenO = 0; writeScreen;}
  wait2 -> Single [order 1] : menuReleased...
      | {screenO = 1; writeScreen;}
  wait1 -> Dual [order 1] : menuReleased...
      | {screenO = 2; writeScreen;}
  data: upTime input uint8; menuTime input uint8; downTime input uint8; startupDelay input double; mode output uint8; x0 output uint8; x1 output uint8; y0 output uint8; y1 output uint8; lineColor output uint8; fillColor output uint8; stringNum output uint8; string output uint8 size=18; font output uint8; FONT4x6 constant uint8 =0; FONT6x8 constant uint8 =1; FONT8x15 constant uint8 =3; WHITE constant uint8 =0; BLACK constant uint8 =1; hCenter output uint8; vCenter output uint8; listIndex input uint8 size=1; singleIndex input double; dualIndex input double; quadIndex input double size=4; screen input uint8; setupNames input double; SETUP_TIME constant uint8 =15; names input uint8; numFields input double; namesline1 input double; namesline2 input double; UPDATE_TIME constant uint16 =2; timer local uint16; oldData local int16 size=6; listIndexO output uint8; barGraphMode input double; barMax input double; barMin input double; temp local int32; screenO output uint8; setupIndex local uint8; setupVIndex local uint8; selectIndex local uint8; selectVIndex local uint8; dualIndexO output uint8 size=2; quadIndexO output uint8 size=4; singleIndexO output uint8; statusTxt input uint8 size=10; statusTxtMode input double; data input int16
  events: tick input EITHER_EDGE_EVENT; setMode output FUNCTION_CALL_EVENT; clearScreen output FUNCTION_CALL_EVENT; drawRect output FUNCTION_CALL_EVENT; drawBitmap output FUNCTION_CALL_EVENT; sendString output FUNCTION_CALL_EVENT; drawString output FUNCTION_CALL_EVENT; drawVLine output FUNCTION_CALL_EVENT; drawHLine output FUNCTION_CALL_EVENT; upPressed input RISING_EDGE_EVENT; upReleased input FALLING_EDGE_EVENT; menuPressed input RISING_EDGE_EVENT; menuReleased input FALLING_EDGE_EVENT; downPressed input RISING_EDGE_EVENT; downReleased input FALLING_EDGE_EVENT; writeListIndex output FUNCTION_CALL_EVENT; writeScreen output FUNCTION_CALL_EVENT; writeDualIndex output FUNCTION_CALL_EVENT; writeSingleIndex output FUNCTION_CALL_EVENT; writeQuadIndex output FUNCTION_CALL_EVENT

== stateflow chart Strategy/MiniViewDisplay/GetFaultName/Chart ==
  state NoFault
    entry:
    text = noErrText;
    during:
    mode = invertMode;
    getNewFault;
  state Fault
    entry:mode = ~invertMode;
    during:minTimer++;
    state scrollText
      entry:
      scrollTimer = 0;
      memcpy(&text[0], &faultName[scrollIndex], dispLength);
      text[dispLength] = uint8(0);
      during:
      scrollTimer++;
    state lastWait
      during:scrollTimer++;
    state scrollTextFirst
      entry:
      scrollTimer = 0;
      scrollIndex = 0;
      minTimer = 0;
      memcpy(&text[0], &faultName[0], dispLength);
      text[dispLength] = uint8(0);
      during:
      scrollTimer++;
    state CheckNextFault
    scrollText -> (junction 359) : [scrollTimer >= scrollTime]
    (junction 359) -> scrollText [order 1] : [faultNameLen-2 >= dispLength+scrollIndex]...
        | {scrollIndex++;}
    (junction 359) -> lastWait [order 2]
    lastWait -> CheckNextFault : [(scrollTimer > lastScrollTime)&&...
        | (minTimer > minTime)]...
        | {getNewFault;}
    (junction 360) -> scrollTextFirst
    (default) -> scrollTextFirst
    scrollTextFirst -> scrollText : [scrollTimer >= firstScrollTime]
        | {scrollIndex++;}
    CheckNextFault -> (junction 361)
    (junction 361) -> (junction 360)
  (default) -> NoFault
  NoFault -> Fault : [faultValid && dispFaults]
  Fault -> NoFault : [~(faultValid && dispFaults)]
  data: invertMode input double; mode output uint8; noErrText input double; text output uint8 size=10; dispLength input double; lastScrollTime input double; scrollTime input double; firstScrollTime input double; dispFaults input double; minTime input double; faultNameLen input double; faultName input double; faultValid input double; minTimer output uint16; scrollIndex output uint8; scrollTimer output uint16
  events: getNewFault output FUNCTION_CALL_EVENT

== matlab function Strategy/MiniViewDisplay/GetFaultName/getStringLength ==
  data: faultName input double; faultNameLength output double
function faultNameLength = fcn(faultName)
% This block supports the Embedded MATLAB subset.
% See the help menu for details. 

faultNameLength = 1;
while((faultName(faultNameLength) ~= 0) ||...
        (faultNameLength > length(faultName)))
    faultNameLength = faultNameLength + 1;
end

== stateflow chart Strategy/Control Strategy/Assist/CruiseControl/Chart ==
  state CruiseDisabled
    entry:state = 0;
    cCOn = 0;
  state CruiseOff
    entry:state = 1;
    cCOn = 0;
  state PressOne
    entry:state = 2;
    timer = 0;
    during:timer++;
  state WaitOne
    entry:state = 3;
    timer = 0;
    during:timer++;
  state PressTwo
    entry:state = 4;
    timer = 0;
    during:timer++;
  state CruiseOn
    entry:state = 5;
    cCOn = 1;
    speedSet = speed;
  CruiseDisabled -> CruiseOff : [cCEnable &&...
      | (speed > minSpeedCC)]
  CruiseOff -> CruiseDisabled [order 1] : [~cCEnable ||...
      | (speed < minSpeedCC)]
  CruiseOff -> PressOne [order 2] : [reverseSw]
  PressOne -> WaitOne [order 2] : [~reverseSw &&...
      |  (timer > minButtonTime)]
  WaitOne -> PressTwo [order 2] : [reverseSw &&...
      |  (timer > minButtonTime)]
  PressTwo -> CruiseOn [order 2] : [~reverseSw &&...
      |  (timer > minButtonTime)]
  PressOne -> (junction 406) [order 1] : [timer > maxButtonTime]
  WaitOne -> (junction 407) [order 1] : [timer > maxButtonTime]
  PressTwo -> (junction 408) [order 1] : [timer > maxButtonTime]
  (junction 408) -> (junction 407)
  (junction 407) -> (junction 406)
  CruiseOn -> (junction 409) : [~cCEnable || cCStop]
  (junction 409) -> (junction 408)
  (junction 406) -> (junction 410)
  (junction 410) -> CruiseOff
  (default) -> CruiseDisabled
  data: reverseSw input double; speed input double; cCEnable input double; cCStop input double; maxButtonTime input double; minButtonTime input double; speedSet output double; cCOn output uint8; state output uint8; timer output uint8; minSpeedCC input double

== stateflow chart Strategy/Actuators/Cruise Control Indicator/Chart ==
  state Off
    entry:light = 0;
  state FlashOne
    entry:light = 1;
    timer = 0;
    during:timer++;
  state FlashTwo
    entry:light = 1;
    timer = 0;
    during:timer++;
  state OffOne
    entry:light = 0;
    timer = 0;
    during:timer++;
  state OffTwo
    entry:light = 0;
    timer = 0;
    during:timer++;
  (default) -> Off
  Off -> FlashOne : [cCOn]
  FlashOne -> OffOne : [timer >= onTime]
  OffOne -> FlashTwo [order 1] : [timer >= offShortTime]
  FlashTwo -> OffTwo : [timer >= onTime]
  OffOne -> (junction 445) [order 2] : [~cCOn]
  OffTwo -> (junction 446) [order 2] : [~cCOn]
  (junction 446) -> (junction 445)
  (junction 445) -> (junction 447)
  (junction 447) -> Off
  (junction 448) -> FlashOne
  OffTwo -> (junction 449) [order 1] : [timer >= offLongTime]
  (junction 449) -> (junction 448)
  data: cCOn input double; light output boolean; offLongTime input double; offShortTime input double; onTime input double; timer local uint16

== stateflow chart Strategy/Control Strategy/ChargeController/Charging State Machine ==
  state Wait
    entry:
    currOut = 0;
    voltOut = 0;
    state = 0;
  state Complete
    entry:
    state = 3;
    currOut = 0;
    voltOut = 0;
  state ConstantVoltageCharge
    entry:
    currOut = CV_CurrentLimit;
    voltOut = CV_Voltage;
    state = 1;
  state waitEnd
    entry:timer = 0;
    state = 2;
    during:timer++;
  state StartupDelay
    entry:state = 4;
    timer = 0;
    during:timer++;
  (default) -> Wait
  StartupDelay -> ConstantVoltageCharge [order 2] : [timer > startupDelay]
  waitEnd -> ConstantVoltageCharge [order 1] : [battCurrent > CV_EndCurrent]
  ConstantVoltageCharge -> waitEnd [order 2] : [battCurrent < CV_EndCurrent]
  waitEnd -> Complete [order 3] : [timer >= CV_EndCurrentTime]
  Wait -> StartupDelay : [startCharge]
  StartupDelay -> Wait [order 1] : [!startCharge]
  ConstantVoltageCharge -> (junction 476) [order 1] : [!startCharge]
  waitEnd -> (junction 477) [order 2] : [!startCharge]
  (junction 477) -> (junction 476)
  (junction 476) -> Wait
  Complete -> (junction 477) : [battVoltage < startChargeVolt]
  data: startCharge input double; battCurrent input double; battVoltage input double; currOut output double; voltOut output double; state output uint8; CV_CurrentLimit input double; CV_EndCurrent input double; CV_Voltage input double; startupDelay input double; timer output uint16; CV_EndCurrentTime input double; startChargeVolt input double

== stateflow chart Strategy/Sensors/Brusa Charger/PluggedInDetect/Chart ==
  state Off
    entry:pluggedIn = 0;
  state countUp
    during:timer++;
  state CountDown
    during:timer--;
  state On
    entry:pluggedIn = 1;
  (default) -> Off
  Off -> countUp : [mainsOn]
  countUp -> CountDown [order 1] : [!mainsOn]
  CountDown -> countUp [order 2] : [mainsOn]
  CountDown -> Off [order 1] : [timer <= 0]
  On -> CountDown : [!mainsOn]
  countUp -> On [order 2] : [timer >= histTime]
  data: histTime input double; mainsOn input double; pluggedIn output boolean; timer local int16
